simulink model "test_libMdl_KalmanFilter"  (R2018a)
settings: Solver=FixedStepAuto  StartTime=0.0  StopTime=200  RelTol=1e-3
PreLoadFcn:
  | init_test_libMdl_KalmanFilter
InitFcn:
  | init_test_libMdl_KalmanFilter
values from neighbouring files (symbols this model uses):
  Q = Gamma*sigma_v^2*Gamma'    [init_test_libMdl_KalmanFilter.m]
  R = sigma_w^2    (= 1)    [init_test_libMdl_KalmanFilter.m]
  sigma_w = 1    [init_test_libMdl_KalmanFilter.m]
  T = 0.5    [init_test_libMdl_KalmanFilter.m]    (also in test_libMdl_KalmanFilter_stateTransitionFcn.m = sample_time)
  x_0 = [50;10]    [init_test_libMdl_KalmanFilter.m]
undefined symbols (not defined in the file or in its folder): mv_seed
libraries: libMdl_KalmanFilter x1, dspsrcs4 x1
settings Model: Creator=hwinter  LastModifiedBy=hwinter

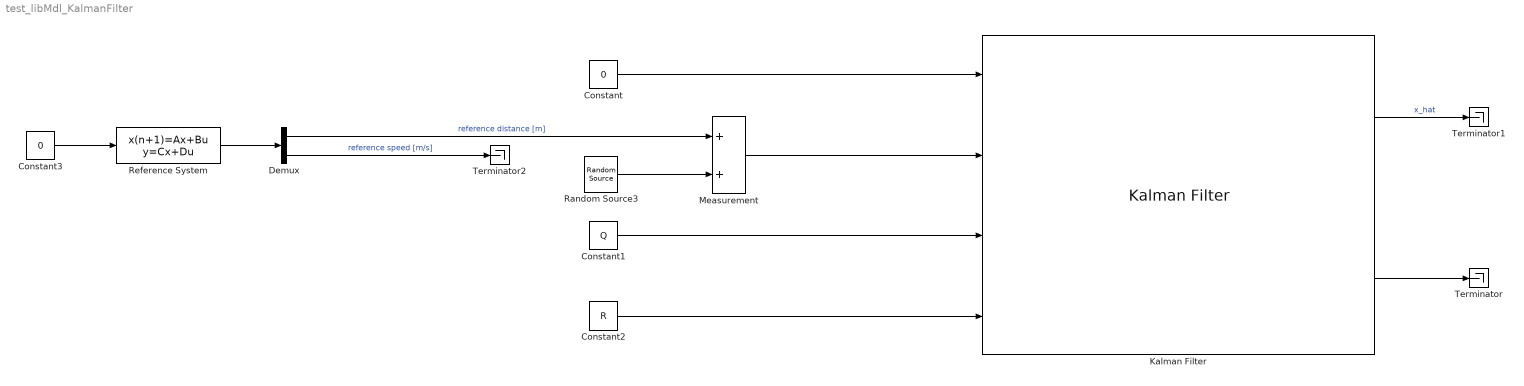
== system test_libMdl_KalmanFilter ==
  Constant : Constant  Value=0
  Constant1 : Constant  Value=Q
  Constant2 : Constant  Value=R
  Constant3 : Constant  Value=0
  Demux : Demux  Outputs=2
  Kalman Filter : libMdl_KalmanFilter/Kalman Filter  mv_sample_time=-1  mv_x_0=x_0  mv_P_0=P_0  mv_state_transition_function=test_libMdl_KalmanFilter_stateTransitionFcn  mv_measurement_function=test_libMdl_KalmanFilter_measurementFcn
  Measurement : Sum
  Random Source3 : dspsrcs4/Random Source  SrcType=Gaussian  NormMethod=Ziggurat  CltLength=12  MinVal=0  MaxVal=1  MeanVal=0  VarVal=sigma_w^2  RepMode=Not repeatable  rawSeed=mv_seed+1  IsInherit=on  SampMode=Discrete  SampTime=1  SampFrame=1  DataType=Double  OutComplex=Real  OutputFrames=off
  Reference System : DiscreteStateSpace  A=[1 T;0 1]  B=[0;0]  C=[1 0;0 1]  D=[0;0]  InitialCondition=x_0  SampleTime=T
  Terminator : Terminator
  Terminator1 : Terminator
  Terminator2 : Terminator
  wires:
  Constant/1 -> Kalman Filter/1
  Measurement/1 -> Kalman Filter/2
  Random Source3/1 -> Measurement/2
  Constant1/1 -> Kalman Filter/3
  Constant2/1 -> Kalman Filter/4
  Kalman Filter/2 -> Terminator/1
  Kalman Filter/1 -> Terminator1/1  "x_hat"
  Constant3/1 -> Reference System/1
  Reference System/1 -> Demux/1
  Demux/1 -> Measurement/1  "reference distance [m]"
  Demux/2 -> Terminator2/1  "reference speed [m/s]"
